simulink model "stateflow1"  (R2015b)
settings: Solver=VariableStepAuto  StartTime=0.0  StopTime=10.0  RelTol=1e-3
libraries: commrandsrc3 x2
settings Model: Creator=etudiant  LastModifiedBy=etudiant

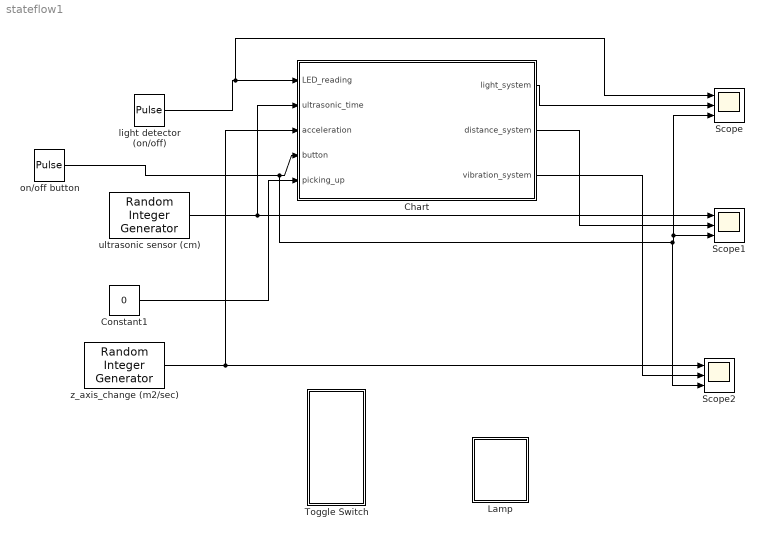
== system stateflow1 ==
  Chart : Stateflow chart  TreatAsAtomicUnit=on
  Constant1 : Constant  Value=0
  Lamp : Subsystem  RequirementInfo="{}  %GIDa_3b593252_faff_4493_aadb_32546510fb03"  DialogController=hmiCreateDDGDialog  IsWebBlock=on  mask(MWDashboardBlock){webBlockId=236d255c-277c-4f79-87dc-d46d00acddbe, webBlockType=lamp, ShowInLibBrowser=on, ShowInitialText=on, HMISrcModelName=stateflow1}
      mask prompts: webBlockType "WebBlock Type"; HMISrcModelName "Source Model"
      mask Help: helpview([docroot '/mapfiles/simulink.map'], 'hmi_lamp')
      mask Display:
      | if strcmp(get_param(bdroot(gcb),'BlockDiagramType'), 'library')
      |     image([(matlabroot) '/toolbox/simulink/hmi/icons/Lamp.png']);
      | end
  Scope : Scope  NumInputPorts=3
  Scope1 : Scope  NumInputPorts=3
  Scope2 : Scope  NumInputPorts=3
  Toggle Switch : Subsystem  DialogController=hmiCreateDDGDialog  IsWebBlock=on  mask(MWDashboardBlock){webBlockId=e06f768c-f5de-466a-8753-f8f2d5380f78, webBlockType=toggleswitch, ShowInLibBrowser=on, ShowInitialText=on, HMISrcModelName=stateflow1}
      mask prompts: webBlockId "WebBlock Id"; webBlockType "WebBlock Type"; HMISrcModelName "Source Model"
      mask Help: helpview([docroot '/mapfiles/simulink.map'], 'hmi_toggle_switch')
      mask Display:
      | if strcmp(get_param(bdroot(gcb),'BlockDiagramType'), 'library')
      |     image([(matlabroot) '/toolbox/simulink/hmi/icons/ToggleSwitch.png']);
      | end
  light detector (on/off) : DiscretePulseGenerator  PulseType=Time based  Period=3  PulseWidth=50
  on/off button : DiscretePulseGenerator  PulseType=Time based  Period=10  PulseWidth=50
  ultrasonic sensor (cm) : commrandsrc3/Random Integer Generator  SetSize=8  SeedSource=Auto  Seed=0  SampleTime=1  SamplesPerFrame=1  OutputDataType=double  SimulateUsing=Interpreted execution
  z_axis_change (m2/sec) : commrandsrc3/Random Integer Generator  SetSize=20  SeedSource=Auto  Seed=0  SampleTime=1  SamplesPerFrame=1  OutputDataType=double  SimulateUsing=Interpreted execution
  wires:
  light detector (on/off)/1 -> Scope/1, Chart/1(LED_reading)
  Chart/1(light_system) -> Scope/2
  Chart/2(distance_system) -> Scope1/2
  ultrasonic sensor (cm)/1 -> Chart/2(ultrasonic_time), Scope1/1
  z_axis_change (m2/sec)/1 -> Scope2/1, Chart/3(acceleration)
  Chart/3(vibration_system) -> Scope2/2
  on/off button/1 -> Scope2/3, Scope1/3, Scope/3, Chart/4(button)
  Constant1/1 -> Chart/5(picking_up)

== system stateflow1/Lamp ==

== system stateflow1/Toggle Switch ==

== stateflow chart stateflow1/Chart ==
  state Power_On
    state dropping_detection [parallel]
      settings: executionOrder=3
      state not_dropped
        entry : t=1;
        during: vibration_system = 0;
      state dropped
        state picked
          entry: adjust_output();
          during: adjust_output();
        state not_picked
          entry: vibration_system =adjust_vibration_intensity(1);;
          during: vibration_system =adjust_vibration_intensity(1);
        (default) -> picked
        picked -> not_picked : [picking_up==0]
        not_picked -> picked : [picking_up==1]
      (default) -> not_dropped
      not_dropped -> dropped : [acceleration >10]
      dropped -> not_dropped : [acceleration<=10]
    state light_detection [parallel]
      settings: executionOrder=1
      state LED_off
        during:light_system=0;
      state LED_on
        during:light_system=1;
      (default) -> LED_off
      LED_off -> LED_on : [LED_reading==1]
      LED_on -> LED_off : [LED_reading==0]
    state distance_detection [parallel]
      during: distance_system = (ultrasonic_time/2) * (340/60);
      settings: executionOrder=2
    (default) -> light_detection
  state Power_off
    during: light_system=0;
    distance_system=0;
    vibration_system=0;
  Power_On -> Power_off : [button==0]
  Power_off -> Power_On : [button==1]
  (default) -> Power_off
  data: a function_input; x function_output; LED_reading input; ultrasonic_time input; light_system output; distance_system output; acceleration input; vibration_system output; button input; t local; picking_up input
  function adjust_output:
    | function adjust_output
    | if t ==1
    | %      pause on;
    |      vibration_system =adjust_vibration_intensity(1);
    | %      pause(0.01);     
    | %      pause off;
    | t=0;
    | else
    |     vibration_system =0;
    |  
    | end    
    |   
    | %     vibration_system =0;
    | 
    | % vibration_system =1;
    | end
  function x=adjust_vibration_intensity(a):
    | function x=adjust_vibration_intensity(a)
    | if a == 1
    | vibration_intensity = mod(((ultrasonic_time/2) * (340/60) ) , 100) + 1; % the intensity is in a scale of 100; the 1 to avoid 0 output
    | else
    |     vibration_intensity = 0;
    | end
    | x = vibration_intensity;
    | end
